simulink model "probl3_lab1"  (Simulink 6.0)
settings: Solver=ode45  StartTime=0.0  StopTime=10.0  RelTol=1e-3
undefined symbols (not defined in the file): kr
libraries: simulink x1
settings Model: LastModifiedBy=student

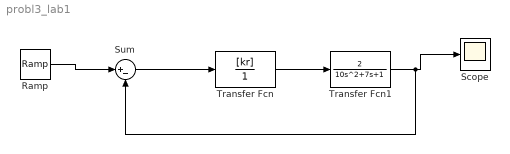
== system probl3_lab1 ==
  Ramp : simulink/Sources/Ramp  slope=1  start=0  X0=0
  Scope : Scope
  Sum : Sum  Inputs=|+-
  Transfer Fcn : TransferFcn  Numerator=[kr]  Denominator=[1]
  Transfer Fcn1 : TransferFcn  Numerator=[2]  Denominator=[10 7 1]
  wires:
  Transfer Fcn1/1 -> Scope/1, Sum/2
  Transfer Fcn/1 -> Transfer Fcn1/1
  Sum/1 -> Transfer Fcn/1
  Ramp/1 -> Sum/1
